simulink model "pll_real"  (R2022a)
settings: Solver=VariableStepAuto  StartTime=0.0  StopTime=10.0  RelTol=1e-3
libraries: spsFirstOrderFilterLib x4, commsynccomp2 x2
settings Model: Creator=fiendchain  LastModifiedBy=fiendchain

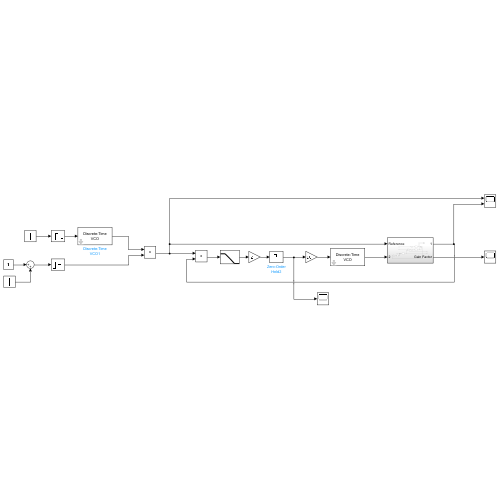
[thumbnail: Simulink's stored preview of the top-level diagram]
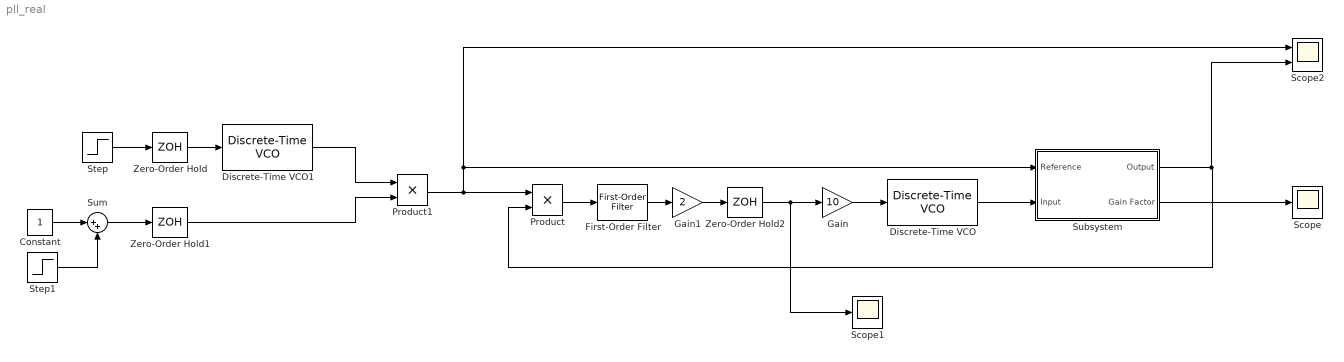
== system pll_real ==
  Constant : Constant
  Discrete-Time VCO : commsynccomp2/Discrete-Time VCO  Ac=1  Fc=50  Kc=1  Ph=0  ts=-1
      settings: SourceProductBaseCode=CM
  Discrete-Time VCO1 : commsynccomp2/Discrete-Time VCO  Ac=1  Fc=50  Kc=1  Ph=0  ts=-1
      settings: SourceProductBaseCode=CM
  First-Order Filter : spsFirstOrderFilterLib/First-Order Filter  FilterType=Lowpass  Tc=1/35  Ts=0  Initialize=on  Vac_Init=[0, 0, 60]  Vdc_Init=0  PlotResponse=off  FreqRange="[0,  200,  1]"
  Gain : Gain  Gain=10
  Gain1 : Gain  Gain=2
  Product : Product
  Product1 : Product
  Scope : Scope
  Scope1 : Scope
  Scope2 : Scope  NumInputPorts=2
  Step : Step  After=-2  SampleTime=0
  Step1 : Step  Time=5  After=0.1  SampleTime=0
  Subsystem : Subsystem
  Sum : Sum  Inputs=|++
  Zero-Order Hold : ZeroOrderHold  SampleTime=1/10000
  Zero-Order Hold1 : ZeroOrderHold  SampleTime=1/10000
  Zero-Order Hold2 : ZeroOrderHold  SampleTime=1/10000
  wires:
  Step/1 -> Zero-Order Hold/1
  Product/1 -> First-Order Filter/1
  First-Order Filter/1 -> Gain1/1
  Product1/1 -> Scope2/1, Subsystem/1(Reference), Product/1
  Discrete-Time VCO/1 -> Subsystem/2(Input)
  Subsystem/1(Output) -> Scope2/2, Product/2
  Discrete-Time VCO1/1 -> Product1/1
  Sum/1 -> Zero-Order Hold1/1
  Constant/1 -> Sum/1
  Step1/1 -> Sum/2
  Subsystem/2(Gain Factor) -> Scope/1
  Zero-Order Hold/1 -> Discrete-Time VCO1/1
  Zero-Order Hold1/1 -> Product1/2
  Zero-Order Hold2/1 -> Gain/1, Scope1/1
  Gain/1 -> Discrete-Time VCO/1
  Gain1/1 -> Zero-Order Hold2/1

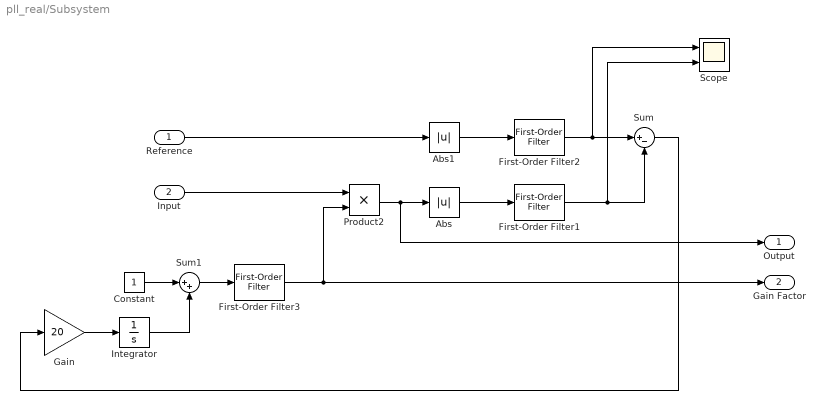
== system pll_real/Subsystem ==
  Reference : Inport
  Input : Inport  Port=2
  Abs : Abs  SaturateOnIntegerOverflow=off
  Abs1 : Abs  SaturateOnIntegerOverflow=off
  Constant : Constant
  First-Order Filter1 : spsFirstOrderFilterLib/First-Order Filter  FilterType=Lowpass  Tc=1/60  Ts=0  Initialize=on  Vac_Init=[0, 0, 60]  Vdc_Init=0  PlotResponse=off  FreqRange="[0,  200,  1]"
  First-Order Filter2 : spsFirstOrderFilterLib/First-Order Filter  FilterType=Lowpass  Tc=1/60  Ts=0  Initialize=on  Vac_Init=[0, 0, 60]  Vdc_Init=0  PlotResponse=off  FreqRange="[0,  200,  1]"
  First-Order Filter3 : spsFirstOrderFilterLib/First-Order Filter  FilterType=Lowpass  Tc=1/100  Ts=0  Initialize=on  Vac_Init=[0, 0, 60]  Vdc_Init=1  PlotResponse=off  FreqRange="[0,  200,  1]"
  Gain : Gain  Gain=20
  Integrator : Integrator  LimitOutput=on  UpperSaturationLimit=0.4  LowerSaturationLimit=-0.4
  Product2 : Product
  Scope : Scope  NumInputPorts=2
  Sum : Sum  Inputs=|+-
  Sum1 : Sum  Inputs=|++
  Output : Outport
  Gain Factor : Outport  Port=2
  wires:
  Product2/1 -> Output/1, Abs/1
  First-Order Filter2/1 -> Sum/1, Scope/1
  Input/1 -> Product2/1
  Sum/1 -> Gain/1
  Reference/1 -> Abs1/1
  Abs/1 -> First-Order Filter1/1
  Abs1/1 -> First-Order Filter2/1
  First-Order Filter1/1 -> Scope/2, Sum/2
  Constant/1 -> Sum1/1
  Gain/1 -> Integrator/1
  Sum1/1 -> First-Order Filter3/1
  Integrator/1 -> Sum1/2
  First-Order Filter3/1 -> Product2/2, Gain Factor/1
